simulink model "j1tb_clctrlDemo"  (R2016b)
settings: Solver=ode5  StartTime=0.0  StopTime=inf  FixedStep=0.001  RelTol=1e-3  EnableMultiTasking=on
undefined symbols (not defined in the file): Humusoft, MF644
libraries: dcpctrl x2, sldrtlib x1
settings Model: SimulationMode=external  Creator=dcp  LastModifiedBy=dcp
settings OptimizationCC: LifeSpan=inf
settings DebuggingCC: SFUnexpectedBacktrackingDiag=warning  SFNoUnconditionalDefaultTransitionDiag=warning  SFExecutionAtInitializationDiag=none
settings HardwareCC: ProdBitPerLong=64  ProdHWDeviceType=Intel->x86-64 (Mac OS X)  TargetBitPerLong=64  TargetBitPerPointer=64  TargetIntDivRoundTo=Zero  TargetEndianess=LittleEndian  TargetWordSize=64  TargetHWDeviceType=Intel->x86-64
settings RTWCC: SystemTargetFile=sldrt.tlc  TemplateMakefile=sldrt.tmf  Description=Simulink Desktop Real-Time  RTWCompilerOptimization=on
settings CodeAppCC: MaxIdLength=95
settings SimulinkDesktopRealTimeCC: TargetPreCompLibLocation=/Applications/MATLAB_R2016b.app/toolbox/sldrt/lib/maci64  TargetLangStandard=C89/C90 (ANSI)  SupportVariableSizeSignals=off
settings ConfigComp: CovMetricSettings=dw  CovHtmlReporting=on  CovSaveCumulativeToWorkspaceVar=on  CovSaveSingleToWorkspaceVar=on  CovExternalEMLEnable=off

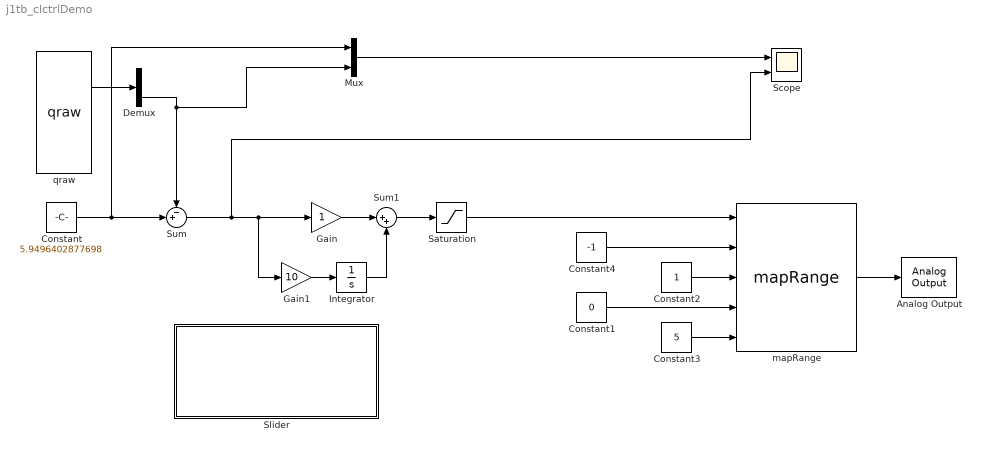
== system j1tb_clctrlDemo ==
  Analog Output : sldrtlib/Analog Output  SampleTime=-1  MaxMissedTicks=10  ShowMissedTicks=off  YieldWhenWaiting=off  DrvName=Humusoft/MF644  DrvAddress=4294967295  DrvOptions=585  Channels=1  RangeMode=1  VoltRange=1  InitialValue=[]  FinalValue=[]
      settings: AttributesFormatString=Humusoft\nMF644 [auto]
  Constant : Constant  Value=5.9496402877698
  Constant1 : Constant  Value=0
  Constant2 : Constant
  Constant3 : Constant  Value=5
  Constant4 : Constant  Value=-1
  Demux : Demux  Outputs=2
  Gain : Gain
  Gain1 : Gain  Gain=10
  Integrator : Integrator  LimitOutput=on  UpperSaturationLimit=1  LowerSaturationLimit=-1
  Mux : Mux  Inputs=2
  Saturation : Saturate  UpperLimit=1  LowerLimit=-1
  Scope : Scope  NumInputPorts=2
  Slider : Subsystem  DialogController=hmiCreateDDGDialog  IsWebBlock=on  mask(MWDashboardBlock){webBlockId=c706c183-58a7-4ae2-9cd4-6a8746b94946, webBlockType=slider, ShowInLibBrowser=on, ShowInitialText=on, HMISrcModelName=j1testbenchclctrlDemo}
      mask prompts: webBlockId "WebBlock Id"; webBlockType "WebBlock Type"; HMISrcModelName "Source Model"
      mask help: SimulinkHMI:dialogs:SliderDialogDesc
      mask Help: helpview([docroot '/mapfiles/simulink.map'], 'hmi_slider')
      mask Display:
      | if strcmp(get_param(bdroot(gcb),'BlockDiagramType'), 'library')
      |     image([(matlabroot) '/toolbox/simulink/hmi/icons/Slider.png']);
      | end
  Sum : Sum  Inputs=-+|
  Sum1 : Sum  Inputs=|++
  "mapRange " : dcpctrl/mapRange 
  qraw : dcpctrl/qraw
  wires:
  "mapRange "/1 -> Analog Output/1
  Constant1/1 -> "mapRange "/4
  Constant2/1 -> "mapRange "/3
  Constant3/1 -> "mapRange "/5
  Constant4/1 -> "mapRange "/2
  qraw/2 -> Demux/1
  Sum/1 -> Scope/2, Gain1/1, Gain/1
  Demux/2 -> Mux/2, Sum/1
  Constant/1 -> Mux/1, Sum/2
  Saturation/1 -> "mapRange "/1
  Mux/1 -> Scope/1
  Integrator/1 -> Sum1/2
  Sum1/1 -> Saturation/1
  Gain/1 -> Sum1/1
  Gain1/1 -> Integrator/1

== system j1tb_clctrlDemo/Slider ==
